simulink model "pid_non_lineare"  (R2021b)
settings: Solver=VariableStepAuto  StartTime=0.0  StopTime=20  RelTol=1e-3
values from neighbouring files (symbols this model uses):
  IC = [0.00 0.00]    [data.m]    (also in postproc2.m = [0.0 0.0])
  PID_sim = PID.v1    [data.m]    (also in postproc2.m = PID(PID_idx(ii)))
  ref = [0.03 0.03]    [data.m]
libraries: slpidlib x2
settings Model: Creator=Daniele Oranges  LastModifiedBy=ernesto

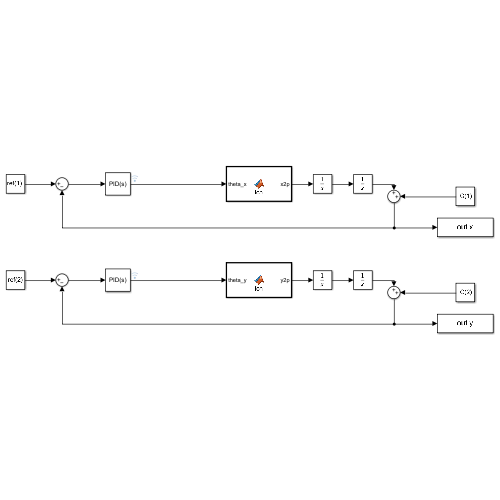
[thumbnail: Simulink's stored preview of the top-level diagram]
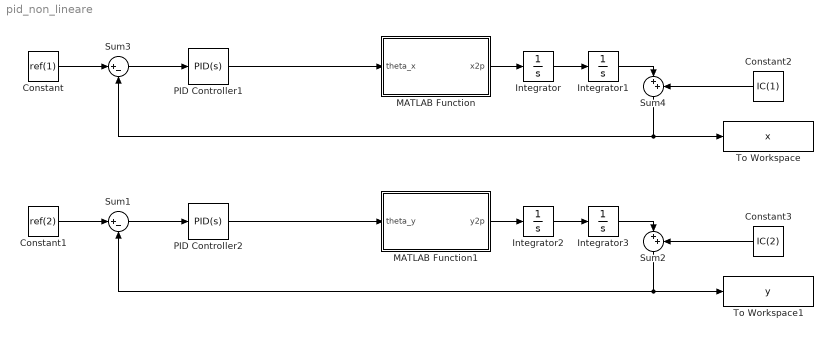
== system pid_non_lineare ==
  Constant : Constant  Value=ref(1)
  Constant1 : Constant  Value=ref(2)
  Constant2 : Constant  Value=IC(1)
  Constant3 : Constant  Value=IC(2)
  Integrator{,1..3} (4 alike) : Integrator
  MATLAB Function : MATLAB Function  TreatAsAtomicUnit=on
  MATLAB Function1 : MATLAB Function  TreatAsAtomicUnit=on
  PID Controller1 : slpidlib/PID Controller  Controller=PID  Form=Parallel  TimeDomain=Continuous-time  UseExternalTs=off  SampleTime=-1  IntegratorMethod=Forward Euler  FilterMethod=Forward Euler  ControllerParametersSource=internal  P=PID_sim.Kp  I=PID_sim.Ki  D=PID_sim.Kd  UseFilter=on  N=PID_sim.filter  TunerSelectOption=Transfer Function Based (PID Tuner App)  InitialConditionSource=internal  InitialConditionForIntegrator=0  InitialConditionForFilter=0  DifferentiatorICPrevScaledInput=0  ExternalReset=none  TrackingMode=off  Kt=1  LimitOutput=off  SatLimitsSource=internal  UpperSaturationLimit=inf  LowerSaturationLimit=-inf  LinearizeAsGain=on  AntiWindupMode=none  Kb=1  POutMin=[]  POutMax=[]  IOutMin=[]  IOutMax=[]  DOutMin=[]  DOutMax=[]  NOutMin=[]  NOutMax=[]  SumOutMin=[]  SumOutMax=[]  SaturationOutMin=[]  SaturationOutMax=[]  PParamMin=[]  PParamMax=[]  IParamMin=[]  IParamMax=[]  DParamMin=[]  DParamMax=[]  NParamMin=[]  NParamMax=[]  KbParamMin=[]  KbParamMax=[]  KtParamMin=[]  KtParamMax=[]  KbOutMin=[]  KbOutMax=[]  KtOutMin=[]  KtOutMax=[]  IntegratorOutMin=[]  IntegratorOutMax=[]  FilterOutMin=[]  FilterOutMax=[]  SumI1OutMin=[]  SumI1OutMax=[]  SumI2OutMin=[]  SumI2OutMax=[]  SumI3OutMin=[]  SumI3OutMax=[]  SumI4OutMin=[]  SumI4OutMax=[]  SumDOutMin=[]  SumDOutMax=[]  DifferentiatorOutMin=[]  DifferentiatorOutMax=[]  FilterDiffOutCoefMin=[]  FilterDiffOutCoefMax=[]  ReciprocalOutMin=[]  ReciprocalOutMax=[]  SumDenOutMin=[]  SumDenOutMax=[]  SumNumOutMin=[]  SumNumOutMax=[]  DivideOutMin=[]  DivideOutMax=[]  UdiffTsProdOutMin=[]  UdiffTsProdOutMax=[]  NTsProdOutMin=[]  NTsProdOutMax=[]  UintegralTsProdOutMin=[]  UintegralTsProdOutMax=[]  UngainTsProdOutMin=[]  UngainTsProdOutMax=[]  IntegratorContinuousStateAttributes=''  IntegratorStateMustResolveToSignalObject=off  IntegratorRTWStateStorageClass=Auto  FilterContinuousStateAttributes=''  FilterStateMustResolveToSignalObject=off  FilterRTWStateStorageClass=Auto  ParallelPVariant=InternalParameters  IdealPVariant=Disabled  IVariant=InternalParameters  DVariant=InternalParameters  IntegratorVariant=Continuous  SatVariant=Disabled  AWVariant=Passthrough  PCopyVariant=Disabled  TRVariant=Disabled  FdbkBlocksVariant=Forward  IdealPFdbkVariant=Disabled  SatFdbkVariant=Disabled  DerivativeFilterVariant=ContFilter  NVariant=InternalParameters  NCopyVariant=Disabled  FilterICVariant=InternalICsFilter  IntegratorICVariant=InternalICs  ExternalResetVariant=Disabled  TRSumVariant=Passthrough  SumFdbkVariant=Disabled  SumVariant=Sum_PID  TsampFilterVariant=InternalTs  TsampNgainVariant=Passthrough  TsampIntegralVariant=Passthrough  ExternalSaturationOutDataTypeStr=Inherit: Same as second input
  PID Controller2 : slpidlib/PID Controller  Controller=PID  Form=Parallel  TimeDomain=Continuous-time  UseExternalTs=off  SampleTime=-1  IntegratorMethod=Forward Euler  FilterMethod=Forward Euler  ControllerParametersSource=internal  P=PID_sim.Kp  I=PID_sim.Ki  D=PID_sim.Kd  UseFilter=on  N=PID_sim.filter  TunerSelectOption=Transfer Function Based (PID Tuner App)  InitialConditionSource=internal  InitialConditionForIntegrator=0  InitialConditionForFilter=0  DifferentiatorICPrevScaledInput=0  ExternalReset=none  TrackingMode=off  Kt=1  LimitOutput=off  SatLimitsSource=internal  UpperSaturationLimit=inf  LowerSaturationLimit=-inf  LinearizeAsGain=on  AntiWindupMode=none  Kb=1  POutMin=[]  POutMax=[]  IOutMin=[]  IOutMax=[]  DOutMin=[]  DOutMax=[]  NOutMin=[]  NOutMax=[]  SumOutMin=[]  SumOutMax=[]  SaturationOutMin=[]  SaturationOutMax=[]  PParamMin=[]  PParamMax=[]  IParamMin=[]  IParamMax=[]  DParamMin=[]  DParamMax=[]  NParamMin=[]  NParamMax=[]  KbParamMin=[]  KbParamMax=[]  KtParamMin=[]  KtParamMax=[]  KbOutMin=[]  KbOutMax=[]  KtOutMin=[]  KtOutMax=[]  IntegratorOutMin=[]  IntegratorOutMax=[]  FilterOutMin=[]  FilterOutMax=[]  SumI1OutMin=[]  SumI1OutMax=[]  SumI2OutMin=[]  SumI2OutMax=[]  SumI3OutMin=[]  SumI3OutMax=[]  SumI4OutMin=[]  SumI4OutMax=[]  SumDOutMin=[]  SumDOutMax=[]  DifferentiatorOutMin=[]  DifferentiatorOutMax=[]  FilterDiffOutCoefMin=[]  FilterDiffOutCoefMax=[]  ReciprocalOutMin=[]  ReciprocalOutMax=[]  SumDenOutMin=[]  SumDenOutMax=[]  SumNumOutMin=[]  SumNumOutMax=[]  DivideOutMin=[]  DivideOutMax=[]  UdiffTsProdOutMin=[]  UdiffTsProdOutMax=[]  NTsProdOutMin=[]  NTsProdOutMax=[]  UintegralTsProdOutMin=[]  UintegralTsProdOutMax=[]  UngainTsProdOutMin=[]  UngainTsProdOutMax=[]  IntegratorContinuousStateAttributes=''  IntegratorStateMustResolveToSignalObject=off  IntegratorRTWStateStorageClass=Auto  FilterContinuousStateAttributes=''  FilterStateMustResolveToSignalObject=off  FilterRTWStateStorageClass=Auto  ParallelPVariant=InternalParameters  IdealPVariant=Disabled  IVariant=InternalParameters  DVariant=InternalParameters  IntegratorVariant=Continuous  SatVariant=Disabled  AWVariant=Passthrough  PCopyVariant=Disabled  TRVariant=Disabled  FdbkBlocksVariant=Forward  IdealPFdbkVariant=Disabled  SatFdbkVariant=Disabled  DerivativeFilterVariant=ContFilter  NVariant=InternalParameters  NCopyVariant=Disabled  FilterICVariant=InternalICsFilter  IntegratorICVariant=InternalICs  ExternalResetVariant=Disabled  TRSumVariant=Passthrough  SumFdbkVariant=Disabled  SumVariant=Sum_PID  TsampFilterVariant=InternalTs  TsampNgainVariant=Passthrough  TsampIntegralVariant=Passthrough  ExternalSaturationOutDataTypeStr=Inherit: Same as second input
  Sum1 : Sum  Inputs=|+-
  Sum2 : Sum  Inputs=|++
  Sum3 : Sum  Inputs=|+-
  Sum4 : Sum  Inputs=|++
  To Workspace : ToWorkspace  VariableName=x  SaveFormat=Timeseries  SampleTime=-1
  To Workspace1 : ToWorkspace  VariableName=y  SaveFormat=Timeseries  SampleTime=-1
  wires:
  Sum3/1 -> PID Controller1/1
  Integrator/1 -> Integrator1/1
  MATLAB Function/1(x2p) -> Integrator/1
  PID Controller1/1 -> MATLAB Function/1(theta_x)
  Sum1/1 -> PID Controller2/1
  PID Controller2/1 -> MATLAB Function1/1(theta_y)
  MATLAB Function1/1(y2p) -> Integrator2/1
  Integrator2/1 -> Integrator3/1
  Sum4/1 -> To Workspace/1, Sum3/2
  Constant3/1 -> Sum2/2
  Constant2/1 -> Sum4/2
  Sum2/1 -> Sum1/2, To Workspace1/1
  Integrator1/1 -> Sum4/1
  Integrator3/1 -> Sum2/1
  Constant1/1 -> Sum1/1
  Constant/1 -> Sum3/1

== matlab function pid_non_lineare/MATLAB Function ==
  data: theta_x input; x2p output
function x2p  = fcn(theta_x)
%% Data

g = 9.81;   % gravitational acceleration [m / s^2]

% Dimensions   [m]
Lx = 0.143;                         % joint position in x direction 
Ly = 0.184;                         % joint position in y direction 
Lx_plane=0.15;                        % plane dimension in x direction 
Ly_plane=0.20 ;                       % plane dimension in y direction      
rm = 0.0245;                        % motor arm length 
lm=0.072 ;                          % motor rod length 
pt = 0.005;                          % plane tickness
d=0.021;                            % plane offset

Mot_Osci_Rang=[-80 ,80];    %(deg)   range di oscilazione dei motori                  
% Ball data                 
rb = 0.02;                          % radius of the ball [m]
mb = 0.265;                         % mass of the ball [kg]
Jb = 0.0000416;                     % rotarional inertia of the ball [kg * m^2]
rho_ball = mb/(4/3 * pi * rb^3);    % ball density [Kg/m^3]


x2p = (mb * g * rb^2 * rm) / ((mb * rb^2 + Jb) * Lx) * sin(theta_x);    % x direction transfer function


end

== matlab function pid_non_lineare/MATLAB Function1 ==
  data: theta_y input; y2p output
function y2p  = fcn(theta_y)
%% Data

g = 9.81;   % gravitational acceleration [m / s^2]

% Dimensions   [m]
Lx = 0.143;                         % joint position in x direction 
Ly = 0.184;                         % joint position in y direction 
Lx_plane=0.15;                        % plane dimension in x direction 
Ly_plane=0.20 ;                       % plane dimension in y direction      
rm = 0.0245;                        % motor arm length 
lm=0.072 ;                          % motor rod length 
pt = 0.005;                          % plane tickness
d=0.021;                            % plane offset

Mot_Osci_Rang=[-80 ,80];    %(deg)   range di oscilazione dei motori                  
% Ball data                 
rb = 0.02;                          % radius of the ball [m]
mb = 0.265;                         % mass of the ball [kg]
Jb = 0.0000416;                     % rotarional inertia of the ball [kg * m^2]
rho_ball = mb/(4/3 * pi * rb^3);    % ball density [Kg/m^3]


y2p = (mb * g * rb^2 * rm) / ((mb * rb^2 + Jb) * Ly) * sin(theta_y);    % x direction transfer function


end
